simulink model "Simulation_adaptive_fuzzy_logic_controller"  (R2023a)
settings: Solver=VariableStepAuto  StartTime=0.0  StopTime=20  RelTol=1e-3
settings Model: Creator=ACCENT  LastModifiedBy=ACCENT

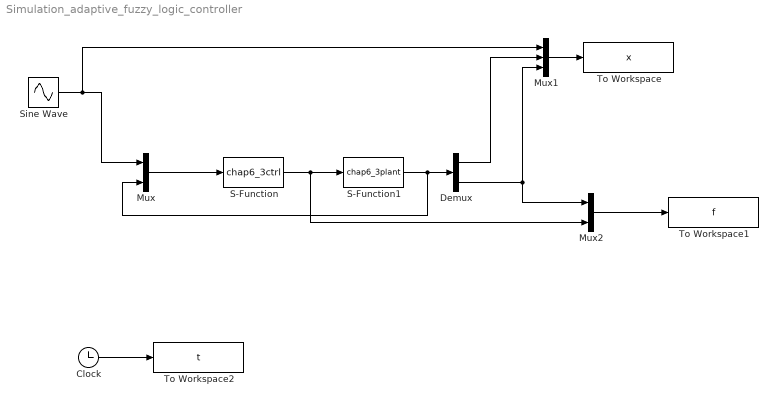
== system Simulation_adaptive_fuzzy_logic_controller ==
  Clock : Clock
      settings: Decimation=20
  Demux : Demux  Outputs=2
  Mux : Mux  Inputs=2
  Mux1 : Mux  Inputs=3
  Mux2 : Mux  Inputs=2
  S-Function : S-Function  FunctionName=chap6_3ctrl  SFunctionDeploymentMode=off  EnableBusSupport=off
  S-Function1 : S-Function  FunctionName=chap6_3plant  SFunctionDeploymentMode=off  EnableBusSupport=off
  Sine Wave : Sin  SampleTime=0
  To Workspace : ToWorkspace  VariableName=x  SampleTime=-1
  To Workspace1 : ToWorkspace  VariableName=f  SampleTime=-1
  To Workspace2 : ToWorkspace  VariableName=t  SampleTime=-1
  wires:
  Sine Wave/1 -> Mux1/1, Mux/1
  Mux/1 -> S-Function/1
  S-Function/1 -> Mux2/2, S-Function1/1
  S-Function1/1 -> Demux/1, Mux/2
  Mux1/1 -> To Workspace/1
  Demux/1 -> Mux1/2
  Demux/2 -> Mux2/1, Mux1/3
  Mux2/1 -> To Workspace1/1
  Clock/1 -> To Workspace2/1
